simulink model "Hopf"  (R2022a)
settings: Solver=VariableStepAuto  StartTime=0.0  StopTime=30  RelTol=1e-3
settings Model: Creator=jandr  LastModifiedBy=jandr

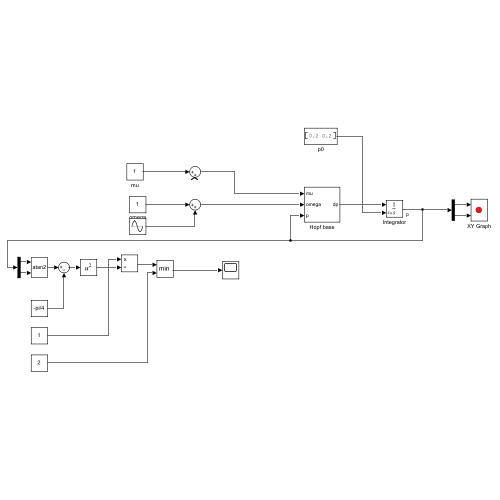
[thumbnail: Simulink's stored preview of the top-level diagram]
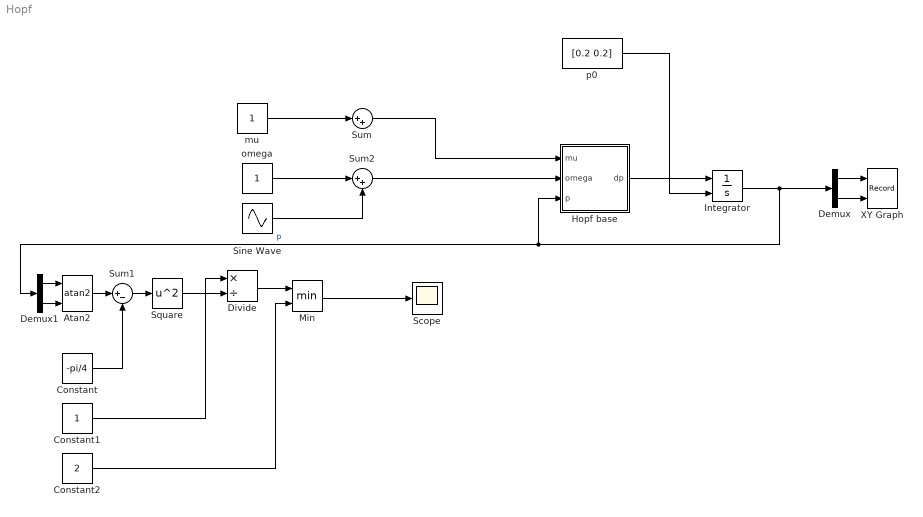
== system Hopf ==
  Atan2 : Trigonometry  Operator=atan2
  Constant : Constant  Value=-pi/4
  Constant1 : Constant
  Constant2 : Constant  Value=2
  Demux : Demux  Outputs=2
  Demux1 : Demux  Outputs=2
  Divide : Product  Inputs=*/
  Hopf base : Subsystem
  Integrator : Integrator  InitialConditionSource=external
  Min : MinMax  Inputs=2
  Scope : Scope
  Sine Wave : Sin  Amplitude=0.5  Frequency=5  SampleTime=0
  Square : Math  Operator=square
  Sum : Sum  Inputs=|++
  Sum1 : Sum  Inputs=|+-
  Sum2 : Sum  Inputs=|++
  XY Graph : Record  FileSettingsInternal="{\"entries\":[{\"content\":{\"excelSettings\":{\"content\":{},\"type\":\"Streamout.ExcelSettings\"}},\"type\":\"Streamout.FileSettingStorage\",\"uuid\":\"5eb4f1f2-ebc8-462a-ba1b-b928507e6297\"}],\"packageUris\":[\"http://schema.mathworks.com/mf0/streamout_blocks/R2020a\"],\"version\":\"1.0\"}"  Layout=[1 1]  SignalsInternal="{\"entries\":[{\"content\":{\"signals\":[{\"content\":{\"blockPath\":[\"Hopf/XY Graph\"],\"channel\":[],\"dimensions\":[1],\"domain\":\"Hopf/XY Graph\",\"lineColor\":\"#a2142f\",\"plots\":[1],\"port\":1,\"sid\":[],\"signalID\":9,\"signalName\":\"Demux:1\"},\"type\":\"RecordBlkView.Signal\",\"uuid\":\"275ea38b-5dc1-4f1b-80bd-5036dce94011\"},{\"content\":{\"blockPath\":[\"Hopf/XY Graph\"],\"channel\":[],\"dimensions\":[1],\"domain\":\"Hopf/XY Graph\",\"lineColor\":\"#139fff\",\"plots\":[1],\"port\":2,\"sid\":[],\"signalID\":12,\"signalName\":\"Demux:2\"},\"type\":\"RecordBlkView.Signal\",\"uuid\":\"97f6d0ee-9d43-4f82-8040-18aa0c9e40f7\"}]},\"type\":\"RecordBlkView.InputSignals\",\"uuid\":\"4cb54163-2614-43d1-8a84-f802e23a08c6\"}],\"packageUris\":[\"http://schema.mathworks.com/mf0/streamout_blocks/R2020a\"],\"version\":\"1.0\"}"  VisualizationBindings="{\"xyplotplugin\":{\"info\":[{\"series\":[{\"bindingParametersList\":[{\"parameter\":\"X-Axis\",\"signalID\":9,\"signalName\":\"Demux:1\"},{\"parameter\":\"Y-Axis\",\"signalID\":12,\"signalName\":\"Demux:2\"}],\"seriesID\":59289}],\"subplotID\":1}]}}"  CompatibilityTag=XY  st=-1
  mu : Constant
  omega : Constant
  p0 : Constant  Value=[0.2 0.2]
  wires:
  p0/1 -> Integrator/2
  Hopf base/1(dp) -> Integrator/1
  Integrator/1 -> Demux/1, Hopf base/3(p), Demux1/1  "p"
  Demux/1 -> XY Graph/1
  Demux/2 -> XY Graph/2
  Sum2/1 -> Hopf base/2(omega)
  Sum/1 -> Hopf base/1(mu)
  mu/1 -> Sum/1
  Demux1/1 -> Atan2/1
  Demux1/2 -> Atan2/2
  Atan2/1 -> Sum1/1
  Sum1/1 -> Square/1
  Constant/1 -> Sum1/2
  Constant1/1 -> Divide/1
  Square/1 -> Divide/2
  Constant2/1 -> Min/2
  Divide/1 -> Min/1
  Min/1 -> Scope/1
  omega/1 -> Sum2/1
  Sine Wave/1 -> Sum2/2

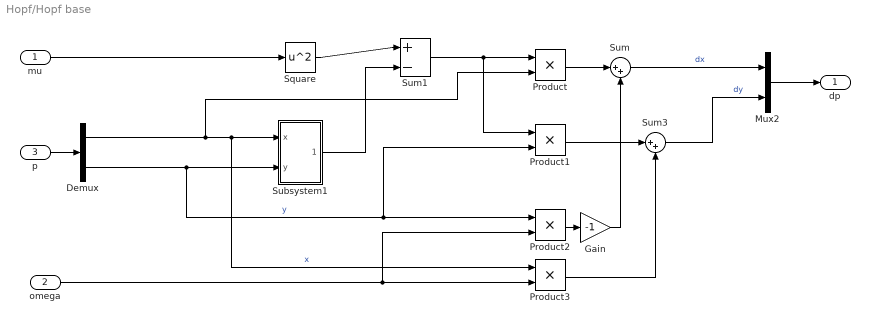
== system Hopf/Hopf base ==
  mu : Inport
  omega : Inport  Port=2
  p : Inport  Port=3
  Demux : Demux  Outputs=2
  Gain : Gain  Gain=-1
  Mux2 : Mux  Inputs=2
  Product{,1..3} (4 alike) : Product
  Square : Math  Operator=square
  Subsystem1 : Subsystem
  Sum : Sum  Inputs=|++
  Sum1 : Sum  Inputs=|+-
  Sum3 : Sum  Inputs=|++
  dp : Outport
  wires:
  Gain/1 -> Sum/2
  Product1/1 -> Sum3/1
  Sum/1 -> Mux2/1  "dx"
  Subsystem1/1(rho2) -> Sum1/2
  Sum1/1 -> Product1/1, Product/1
  mu/1 -> Square/1
  Product/1 -> Sum/1
  Sum3/1 -> Mux2/2  "dy"
  Mux2/1 -> dp/1
  p/1 -> Demux/1
  Demux/1 -> Product/2, Product3/1, Subsystem1/1(x)  "x"
  Demux/2 -> Product2/1, Product1/2, Subsystem1/2(y)  "y"
  Square/1 -> Sum1/1
  Product2/1 -> Gain/1
  Product3/1 -> Sum3/2
  omega/1 -> Product2/2, Product3/2

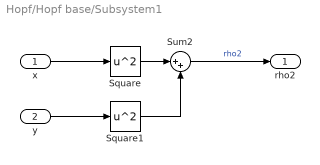
== system Hopf/Hopf base/Subsystem1 ==
  x : Inport
  y : Inport  Port=2
  Square : Math  Operator=square
  Square1 : Math  Operator=square
  Sum2 : Sum  Inputs=|++
  rho2 : Outport
  wires:
  Square/1 -> Sum2/1
  Sum2/1 -> rho2/1  "rho2"
  Square1/1 -> Sum2/2
  x/1 -> Square/1
  y/1 -> Square1/1
